simulink model "master_thesis_simulink"  (R2022a)
settings: Solver=VariableStepAuto  StartTime=0.0  StopTime=p_0p.time(end)  FixedStep=0.001  RelTol=1e-3
values from neighbouring files (symbols this model uses):
  markers_forearm = [0.00210510253906 -0.143263397217 -0.00798474121094]    [markers_forearm.mat]
  markers_shoulder = [0.010127746582 -0.151647644043 -0.0119686279297]    [markers_shoulder.mat]
undefined symbols (not defined in the file or in its folder): arm, DiscIntNeverNeededParam, Discrete, ekf, kf, LS, m, markers_hand, n, noise, q0, q0_LS, q0_model, sample_Time, selected, state_observer, Time, tSh_0_0Conf, X, Y, Z
libraries: sm_lib x2029, nesl_utility x1553, robotlib x75, ctrlSharedLib x8
(part 33 of 70)

== system master_thesis_simulink/Ros2Matlab/S1_F1_H2/Subscriber/M3/Pose ==
  Bus : BusSelector  OutputSignals=Pose.Position.X,Pose.Position.Y,Pose.Position.Z
  Mux : Mux  Inputs=3
  Subscribe_pose : robotlib/Subscribe  topicSource=Select from ROS network  topic=/qualisys/Super_marker_3/pose  messageType=geometry_msgs/PoseStamped  SampleTime=sample_Time  legacyBusStruct=off  messageQueueLength=1
  p3_W : Outport
  tag scope: M3_isNew=global
  wires:
  Bus/1 -> Mux/1  "<X>"
  Mux/1 -> p3_W/1
  Subscribe_pose/2 -> Bus/1
  Bus/3 -> Mux/3  "<Z>"
  Bus/2 -> Mux/2  "<Y>"
  Subscribe_pose/1 -> [M3_isNew]

== system master_thesis_simulink/Ros2Matlab/S1_F1_H2/Subscriber/M4/Odom ==
  Bus1 : BusSelector  OutputSignals=Twist.Twist.Linear.X,Twist.Twist.Linear.Y,Twist.Twist.Linear.Z
  Bus2 : BusSelector  OutputSignals=Pose.Covariance
  Bus3 : BusSelector  OutputSignals=Twist.Covariance
  Mux2 : Mux  Inputs=3
  Subscribe_twist : robotlib/Subscribe  topicSource=Select from ROS network  topic=/qualisys/Super_marker_4/odom  messageType=nav_msgs/Odometry  SampleTime=sample_Time  legacyBusStruct=off  messageQueueLength=1
  Terminator3 : Terminator
  v4_W : Outport
  Rp4_W : Outport  Port=2
  Rv4_W : Outport  Port=3
  wires:
  Mux2/1 -> v4_W/1
  Subscribe_twist/1 -> Terminator3/1
  Bus1/2 -> Mux2/2  "<Y>"
  Bus1/1 -> Mux2/1  "<X>"
  Bus1/3 -> Mux2/3  "<Z>"
  Subscribe_twist/2 -> Bus3/1, Bus2/1, Bus1/1
  Bus2/1 -> Rp4_W/1  "<Covariance>"
  Bus3/1 -> Rv4_W/1  "<Covariance>"

== system master_thesis_simulink/Ros2Matlab/S1_F1_H2/Subscriber/M4/Pose ==
  Bus : BusSelector  OutputSignals=Pose.Position.X,Pose.Position.Y,Pose.Position.Z
  Mux : Mux  Inputs=3
  Subscribe_pose : robotlib/Subscribe  topicSource=Select from ROS network  topic=/qualisys/Super_marker_4/pose  messageType=geometry_msgs/PoseStamped  SampleTime=sample_Time  legacyBusStruct=off  messageQueueLength=1
  p4_W : Outport
  tag scope: M4_isNew=global
  wires:
  Bus/2 -> Mux/2  "<Y>"
  Bus/3 -> Mux/3  "<Z>"
  Subscribe_pose/2 -> Bus/1
  Mux/1 -> p4_W/1
  Bus/1 -> Mux/1  "<X>"
  Subscribe_pose/1 -> [M4_isNew]

== system master_thesis_simulink/Ros2Matlab/S1_F1_H2/Subscriber/Shoulder_RF/Pose ==
  Bus Selector : BusSelector  OutputSignals=Pose.Orientation.W
  Bus Selector1 : BusSelector  OutputSignals=Pose.Orientation.X
  Bus Selector2 : BusSelector  OutputSignals=Pose.Orientation.Y
  Bus Selector3 : BusSelector  OutputSignals=Pose.Position.X,Pose.Position.Y,Pose.Position.Z
  Bus Selector4 : BusSelector  OutputSignals=Pose.Orientation.Z
  Mux1 : Mux  Inputs=3
  Mux2 : Mux
  Subscribe_pose : robotlib/Subscribe  topicSource=Select from ROS network  topic=/qualisys/Shoulder_RF/pose  messageType=geometry_msgs/PoseStamped  SampleTime=sample_Time  legacyBusStruct=off  messageQueueLength=1
  quat_Sh2W : Outport
  pSh_W : Outport  Port=2
  tag scope: Sh_isNew=global
  wires:
  Mux2/1 -> quat_Sh2W/1
  Bus Selector4/1 -> Mux2/4  "<Z>"
  Mux1/1 -> pSh_W/1
  Bus Selector3/3 -> Mux1/3  "<Z>"
  Bus Selector3/2 -> Mux1/2  "<Y>"
  Bus Selector3/1 -> Mux1/1  "<X>"
  Bus Selector2/1 -> Mux2/3  "<Y>"
  Bus Selector1/1 -> Mux2/2  "<X>"
  Bus Selector/1 -> Mux2/1  "<W>"
  Subscribe_pose/2 -> Bus Selector/1, Bus Selector1/1, Bus Selector2/1, Bus Selector3/1, Bus Selector4/1
  Subscribe_pose/1 -> [Sh_isNew]

== system master_thesis_simulink/Ros2Matlab/S1_F2_H2/Subscriber/M0/Odom ==
  Bus Selector : BusSelector  OutputSignals=Pose.Covariance
  Bus Selector1 : BusSelector  OutputSignals=Twist.Covariance
  Bus1 : BusSelector  OutputSignals=Twist.Twist.Linear.X,Twist.Twist.Linear.Y,Twist.Twist.Linear.Z
  Mux2 : Mux  Inputs=3
  Subscribe_odom : robotlib/Subscribe  topicSource=Select from ROS network  topic=/qualisys/Super_marker_0/odom  messageType=nav_msgs/Odometry  SampleTime=sample_Time  legacyBusStruct=off  messageQueueLength=1
  Terminator3 : Terminator
  v0_W : Outport
  Rp0_W : Outport  Port=2
  Rv0_W : Outport  Port=3
  wires:
  Bus Selector1/1 -> Rv0_W/1  "<Covariance>"
  Bus Selector/1 -> Rp0_W/1  "<Covariance>"
  Subscribe_odom/2 -> Bus1/1, Bus Selector/1, Bus Selector1/1
  Mux2/1 -> v0_W/1
  Subscribe_odom/1 -> Terminator3/1
  Bus1/2 -> Mux2/2  "<Y>"
  Bus1/1 -> Mux2/1  "<X>"
  Bus1/3 -> Mux2/3  "<Z>"

== system master_thesis_simulink/Ros2Matlab/S1_F2_H2/Subscriber/M0/Pose ==
  Bus Selector : BusSelector  OutputSignals=Pose.Orientation.W
  Bus Selector1 : BusSelector  OutputSignals=Pose.Orientation.X
  Bus Selector2 : BusSelector  OutputSignals=Pose.Orientation.Y
  Bus Selector3 : BusSelector  OutputSignals=Pose.Position.X,Pose.Position.Y,Pose.Position.Z
  Bus Selector4 : BusSelector  OutputSignals=Pose.Orientation.Z
  Mux1 : Mux  Inputs=3
  Mux2 : Mux
  Subscribe_pose : robotlib/Subscribe  topicSource=Select from ROS network  topic=/qualisys/Super_marker_0/pose  messageType=geometry_msgs/PoseStamped  SampleTime=sample_Time  legacyBusStruct=off  messageQueueLength=1
  quat_02W : Outport
  p0_W : Outport  Port=2
  tag scope: M0_isNew=global
  wires:
  Subscribe_pose/1 -> [M0_isNew]
  Subscribe_pose/2 -> Bus Selector4/1, Bus Selector3/1, Bus Selector2/1, Bus Selector1/1, Bus Selector/1
  Bus Selector/1 -> Mux2/1  "<W>"
  Bus Selector1/1 -> Mux2/2  "<X>"
  Bus Selector2/1 -> Mux2/3  "<Y>"
  Bus Selector3/1 -> Mux1/1  "<X>"
  Bus Selector3/2 -> Mux1/2  "<Y>"
  Bus Selector3/3 -> Mux1/3  "<Z>"
  Mux1/1 -> p0_W/1
  Bus Selector4/1 -> Mux2/4  "<Z>"
  Mux2/1 -> quat_02W/1

== system master_thesis_simulink/Ros2Matlab/S1_F2_H2/Subscriber/M1/Odom ==
  Bus1 : BusSelector  OutputSignals=Twist.Twist.Linear.X,Twist.Twist.Linear.Y,Twist.Twist.Linear.Z
  Bus2 : BusSelector  OutputSignals=Pose.Covariance
  Bus3 : BusSelector  OutputSignals=Twist.Covariance
  Mux2 : Mux  Inputs=3
  Subscribe_twist : robotlib/Subscribe  topicSource=Select from ROS network  topic=/qualisys/Super_marker_1/odom  messageType=nav_msgs/Odometry  SampleTime=sample_Time  legacyBusStruct=off  messageQueueLength=1
  Terminator3 : Terminator
  v1_W : Outport
  Rp1_W : Outport  Port=2
  Rv1_W : Outport  Port=3
  wires:
  Bus3/1 -> Rv1_W/1  "<Covariance>"
  Bus2/1 -> Rp1_W/1  "<Covariance>"
  Subscribe_twist/2 -> Bus1/1, Bus2/1, Bus3/1
  Mux2/1 -> v1_W/1
  Subscribe_twist/1 -> Terminator3/1
  Bus1/2 -> Mux2/2  "<Y>"
  Bus1/1 -> Mux2/1  "<X>"
  Bus1/3 -> Mux2/3  "<Z>"

== system master_thesis_simulink/Ros2Matlab/S1_F2_H2/Subscriber/M1/Pose ==
  Bus : BusSelector  OutputSignals=Pose.Position.X,Pose.Position.Y,Pose.Position.Z
  Mux : Mux  Inputs=3
  Subscribe_pose : robotlib/Subscribe  topicSource=Select from ROS network  topic=/qualisys/Super_marker_1/pose  messageType=geometry_msgs/PoseStamped  SampleTime=sample_Time  legacyBusStruct=off  messageQueueLength=1
  p1_W : Outport
  tag scope: M1_isNew=global
  wires:
  Subscribe_pose/1 -> [M1_isNew]
  Bus/2 -> Mux/2  "<Y>"
  Bus/3 -> Mux/3  "<Z>"
  Subscribe_pose/2 -> Bus/1
  Mux/1 -> p1_W/1
  Bus/1 -> Mux/1  "<X>"

== system master_thesis_simulink/Ros2Matlab/S1_F2_H2/Subscriber/M2/Odom ==
  Bus1 : BusSelector  OutputSignals=Twist.Twist.Linear.X,Twist.Twist.Linear.Y,Twist.Twist.Linear.Z
  Bus2 : BusSelector  OutputSignals=Pose.Covariance
  Bus3 : BusSelector  OutputSignals=Twist.Covariance
  Mux2 : Mux  Inputs=3
  Subscribe_twist : robotlib/Subscribe  topicSource=Select from ROS network  topic=/qualisys/Super_marker_2/odom  messageType=nav_msgs/Odometry  SampleTime=sample_Time  legacyBusStruct=off  messageQueueLength=1
  Terminator3 : Terminator
  v2_W : Outport
  Rp2_W : Outport  Port=2
  Rv2_W : Outport  Port=3
  wires:
  Bus3/1 -> Rv2_W/1  "<Covariance>"
  Subscribe_twist/2 -> Bus1/1, Bus2/1, Bus3/1
  Bus2/1 -> Rp2_W/1  "<Covariance>"
  Bus1/3 -> Mux2/3  "<Z>"
  Bus1/1 -> Mux2/1  "<X>"
  Bus1/2 -> Mux2/2  "<Y>"
  Subscribe_twist/1 -> Terminator3/1
  Mux2/1 -> v2_W/1

== system master_thesis_simulink/Ros2Matlab/S1_F2_H2/Subscriber/M2/Pose ==
  Bus : BusSelector  OutputSignals=Pose.Position.X,Pose.Position.Y,Pose.Position.Z
  Mux : Mux  Inputs=3
  Subscribe_pose : robotlib/Subscribe  topicSource=Select from ROS network  topic=/qualisys/Super_marker_2/pose  messageType=geometry_msgs/PoseStamped  SampleTime=sample_Time  legacyBusStruct=off  messageQueueLength=1
  p2_W : Outport
  tag scope: M2_isNew=global
  wires:
  Subscribe_pose/1 -> [M2_isNew]
  Bus/1 -> Mux/1  "<X>"
  Mux/1 -> p2_W/1
  Subscribe_pose/2 -> Bus/1
  Bus/3 -> Mux/3  "<Z>"
  Bus/2 -> Mux/2  "<Y>"

== system master_thesis_simulink/Ros2Matlab/S1_F2_H2/Subscriber/M3/Odom ==
  Bus1 : BusSelector  OutputSignals=Twist.Twist.Linear.X,Twist.Twist.Linear.Y,Twist.Twist.Linear.Z
  Bus2 : BusSelector  OutputSignals=Pose.Covariance
  Bus3 : BusSelector  OutputSignals=Twist.Covariance
  Mux2 : Mux  Inputs=3
  Subscribe_twist : robotlib/Subscribe  topicSource=Select from ROS network  topic=/qualisys/Super_marker_3/odom  messageType=nav_msgs/Odometry  SampleTime=sample_Time  legacyBusStruct=off  messageQueueLength=1
  Terminator3 : Terminator
  v3_W : Outport
  Rp3_W : Outport  Port=2
  Rv3_W : Outport  Port=3
  wires:
  Bus3/1 -> Rv3_W/1  "<Covariance>"
  Subscribe_twist/2 -> Bus1/1, Bus2/1, Bus3/1
  Bus2/1 -> Rp3_W/1  "<Covariance>"
  Mux2/1 -> v3_W/1
  Subscribe_twist/1 -> Terminator3/1
  Bus1/2 -> Mux2/2  "<Y>"
  Bus1/1 -> Mux2/1  "<X>"
  Bus1/3 -> Mux2/3  "<Z>"

== system master_thesis_simulink/Ros2Matlab/S1_F2_H2/Subscriber/M3/Pose ==
  Bus : BusSelector  OutputSignals=Pose.Position.X,Pose.Position.Y,Pose.Position.Z
  Mux : Mux  Inputs=3
  Subscribe_pose : robotlib/Subscribe  topicSource=Select from ROS network  topic=/qualisys/Super_marker_3/pose  messageType=geometry_msgs/PoseStamped  SampleTime=sample_Time  legacyBusStruct=off  messageQueueLength=1
  p3_W : Outport
  tag scope: M3_isNew=global
  wires:
  Subscribe_pose/1 -> [M3_isNew]
  Bus/2 -> Mux/2  "<Y>"
  Bus/3 -> Mux/3  "<Z>"
  Subscribe_pose/2 -> Bus/1
  Mux/1 -> p3_W/1
  Bus/1 -> Mux/1  "<X>"

== system master_thesis_simulink/Ros2Matlab/S1_F2_H2/Subscriber/M4/Odom ==
  Bus1 : BusSelector  OutputSignals=Twist.Twist.Linear.X,Twist.Twist.Linear.Y,Twist.Twist.Linear.Z
  Bus2 : BusSelector  OutputSignals=Pose.Covariance
  Bus3 : BusSelector  OutputSignals=Twist.Covariance
  Mux2 : Mux  Inputs=3
  Subscribe_twist : robotlib/Subscribe  topicSource=Select from ROS network  topic=/qualisys/Super_marker_4/odom  messageType=nav_msgs/Odometry  SampleTime=sample_Time  legacyBusStruct=off  messageQueueLength=1
  Terminator3 : Terminator
  v4_W : Outport
  Rp4_W : Outport  Port=2
  Rv4_W : Outport  Port=3
  wires:
  Bus3/1 -> Rv4_W/1  "<Covariance>"
  Bus2/1 -> Rp4_W/1  "<Covariance>"
  Subscribe_twist/2 -> Bus1/1, Bus2/1, Bus3/1
  Bus1/3 -> Mux2/3  "<Z>"
  Bus1/1 -> Mux2/1  "<X>"
  Bus1/2 -> Mux2/2  "<Y>"
  Subscribe_twist/1 -> Terminator3/1
  Mux2/1 -> v4_W/1

== system master_thesis_simulink/Ros2Matlab/S1_F2_H2/Subscriber/M4/Pose ==
  Bus : BusSelector  OutputSignals=Pose.Position.X,Pose.Position.Y,Pose.Position.Z
  Mux : Mux  Inputs=3
  Subscribe_pose : robotlib/Subscribe  topicSource=Select from ROS network  topic=/qualisys/Super_marker_4/pose  messageType=geometry_msgs/PoseStamped  SampleTime=sample_Time  legacyBusStruct=off  messageQueueLength=1
  p4_W : Outport
  tag scope: M4_isNew=global
  wires:
  Subscribe_pose/1 -> [M4_isNew]
  Bus/1 -> Mux/1  "<X>"
  Mux/1 -> p4_W/1
  Subscribe_pose/2 -> Bus/1
  Bus/3 -> Mux/3  "<Z>"
  Bus/2 -> Mux/2  "<Y>"

== system master_thesis_simulink/Ros2Matlab/S1_F2_H2/Subscriber/M5/Odom ==
  Bus1 : BusSelector  OutputSignals=Twist.Twist.Linear.X,Twist.Twist.Linear.Y,Twist.Twist.Linear.Z
  Bus2 : BusSelector  OutputSignals=Pose.Covariance
  Bus3 : BusSelector  OutputSignals=Twist.Covariance
  Mux2 : Mux  Inputs=3
  Subscribe_twist : robotlib/Subscribe  topicSource=Select from ROS network  topic=/qualisys/Super_marker_5/odom  messageType=nav_msgs/Odometry  SampleTime=sample_Time  legacyBusStruct=off  messageQueueLength=1
  Terminator3 : Terminator
  v2_W : Outport
  Rp2_W : Outport  Port=2
  Rv2_W : Outport  Port=3
  wires:
  Mux2/1 -> v2_W/1
  Subscribe_twist/1 -> Terminator3/1
  Bus1/2 -> Mux2/2  "<Y>"
  Bus1/1 -> Mux2/1  "<X>"
  Bus1/3 -> Mux2/3  "<Z>"
  Bus2/1 -> Rp2_W/1  "<Covariance>"
  Subscribe_twist/2 -> Bus3/1, Bus2/1, Bus1/1
  Bus3/1 -> Rv2_W/1  "<Covariance>"

== system master_thesis_simulink/Ros2Matlab/S1_F2_H2/Subscriber/M5/Pose ==
  Bus : BusSelector  OutputSignals=Pose.Position.X,Pose.Position.Y,Pose.Position.Z
  Mux : Mux  Inputs=3
  Subscribe_pose : robotlib/Subscribe  topicSource=Select from ROS network  topic=/qualisys/Super_marker_5/pose  messageType=geometry_msgs/PoseStamped  SampleTime=sample_Time  legacyBusStruct=off  messageQueueLength=1
  p5_W : Outport
  tag scope: M5_isNew=global
  wires:
  Bus/2 -> Mux/2  "<Y>"
  Bus/3 -> Mux/3  "<Z>"
  Subscribe_pose/2 -> Bus/1
  Mux/1 -> p5_W/1
  Bus/1 -> Mux/1  "<X>"
  Subscribe_pose/1 -> [M5_isNew]

== system master_thesis_simulink/Ros2Matlab/S1_F2_H2/Subscriber/Shoulder_RF/Pose ==
  Bus Selector : BusSelector  OutputSignals=Pose.Orientation.W
  Bus Selector1 : BusSelector  OutputSignals=Pose.Orientation.X
  Bus Selector2 : BusSelector  OutputSignals=Pose.Orientation.Y
  Bus Selector3 : BusSelector  OutputSignals=Pose.Position.X,Pose.Position.Y,Pose.Position.Z
  Bus Selector4 : BusSelector  OutputSignals=Pose.Orientation.Z
  Mux1 : Mux  Inputs=3
  Mux2 : Mux
  Subscribe_pose : robotlib/Subscribe  topicSource=Select from ROS network  topic=/qualisys/Shoulder_RF/pose  messageType=geometry_msgs/PoseStamped  SampleTime=sample_Time  legacyBusStruct=off  messageQueueLength=1
  quat_Sh2W : Outport
  pSh_W : Outport  Port=2
  tag scope: Sh_isNew=global
  wires:
  Subscribe_pose/1 -> [Sh_isNew]
  Subscribe_pose/2 -> Bus Selector4/1, Bus Selector3/1, Bus Selector2/1, Bus Selector1/1, Bus Selector/1
  Bus Selector/1 -> Mux2/1  "<W>"
  Bus Selector1/1 -> Mux2/2  "<X>"
  Bus Selector2/1 -> Mux2/3  "<Y>"
  Bus Selector3/1 -> Mux1/1  "<X>"
  Bus Selector3/2 -> Mux1/2  "<Y>"
  Bus Selector3/3 -> Mux1/3  "<Z>"
  Mux1/1 -> pSh_W/1
  Bus Selector4/1 -> Mux2/4  "<Z>"
  Mux2/1 -> quat_Sh2W/1

== system master_thesis_simulink/Ros2Matlab/S2_F0_H2/Subscriber/M0/Odom ==
  Bus Selector : BusSelector  OutputSignals=Pose.Covariance
  Bus Selector1 : BusSelector  OutputSignals=Twist.Covariance
  Bus1 : BusSelector  OutputSignals=Twist.Twist.Linear.X,Twist.Twist.Linear.Y,Twist.Twist.Linear.Z
  Mux2 : Mux  Inputs=3
  Subscribe_odom : robotlib/Subscribe  topicSource=Select from ROS network  topic=/qualisys/Super_marker_0/odom  messageType=nav_msgs/Odometry  SampleTime=sample_Time  legacyBusStruct=off  messageQueueLength=1
  Terminator3 : Terminator
  v0_W : Outport
  Rp0_W : Outport  Port=2
  Rv0_W : Outport  Port=3
  wires:
  Bus1/3 -> Mux2/3  "<Z>"
  Bus1/1 -> Mux2/1  "<X>"
  Bus1/2 -> Mux2/2  "<Y>"
  Subscribe_odom/1 -> Terminator3/1
  Mux2/1 -> v0_W/1
  Subscribe_odom/2 -> Bus Selector1/1, Bus Selector/1, Bus1/1
  Bus Selector/1 -> Rp0_W/1  "<Covariance>"
  Bus Selector1/1 -> Rv0_W/1  "<Covariance>"

== system master_thesis_simulink/Ros2Matlab/S2_F0_H2/Subscriber/M0/Pose ==
  Bus Selector : BusSelector  OutputSignals=Pose.Orientation.W
  Bus Selector1 : BusSelector  OutputSignals=Pose.Orientation.X
  Bus Selector2 : BusSelector  OutputSignals=Pose.Orientation.Y
  Bus Selector3 : BusSelector  OutputSignals=Pose.Position.X,Pose.Position.Y,Pose.Position.Z
  Bus Selector4 : BusSelector  OutputSignals=Pose.Orientation.Z
  Mux1 : Mux  Inputs=3
  Mux2 : Mux
  Subscribe_pose : robotlib/Subscribe  topicSource=Select from ROS network  topic=/qualisys/Super_marker_0/pose  messageType=geometry_msgs/PoseStamped  SampleTime=sample_Time  legacyBusStruct=off  messageQueueLength=1
  quat_02W : Outport
  p0_W : Outport  Port=2
  tag scope: M0_isNew=global
  wires:
  Mux2/1 -> quat_02W/1
  Bus Selector4/1 -> Mux2/4  "<Z>"
  Mux1/1 -> p0_W/1
  Bus Selector3/3 -> Mux1/3  "<Z>"
  Bus Selector3/2 -> Mux1/2  "<Y>"
  Bus Selector3/1 -> Mux1/1  "<X>"
  Bus Selector2/1 -> Mux2/3  "<Y>"
  Bus Selector1/1 -> Mux2/2  "<X>"
  Bus Selector/1 -> Mux2/1  "<W>"
  Subscribe_pose/2 -> Bus Selector/1, Bus Selector1/1, Bus Selector2/1, Bus Selector3/1, Bus Selector4/1
  Subscribe_pose/1 -> [M0_isNew]

== system master_thesis_simulink/Ros2Matlab/S2_F0_H2/Subscriber/M1/Odom ==
  Bus1 : BusSelector  OutputSignals=Twist.Twist.Linear.X,Twist.Twist.Linear.Y,Twist.Twist.Linear.Z
  Bus2 : BusSelector  OutputSignals=Pose.Covariance
  Bus3 : BusSelector  OutputSignals=Twist.Covariance
  Mux2 : Mux  Inputs=3
  Subscribe_twist : robotlib/Subscribe  topicSource=Select from ROS network  topic=/qualisys/Super_marker_1/odom  messageType=nav_msgs/Odometry  SampleTime=sample_Time  legacyBusStruct=off  messageQueueLength=1
  Terminator3 : Terminator
  v1_W : Outport
  Rp1_W : Outport  Port=2
  Rv1_W : Outport  Port=3
  wires:
  Bus1/3 -> Mux2/3  "<Z>"
  Bus1/1 -> Mux2/1  "<X>"
  Bus1/2 -> Mux2/2  "<Y>"
  Subscribe_twist/1 -> Terminator3/1
  Mux2/1 -> v1_W/1
  Subscribe_twist/2 -> Bus3/1, Bus2/1, Bus1/1
  Bus2/1 -> Rp1_W/1  "<Covariance>"
  Bus3/1 -> Rv1_W/1  "<Covariance>"

== system master_thesis_simulink/Ros2Matlab/S2_F0_H2/Subscriber/M1/Pose ==
  Bus : BusSelector  OutputSignals=Pose.Position.X,Pose.Position.Y,Pose.Position.Z
  Mux : Mux  Inputs=3
  Subscribe_pose : robotlib/Subscribe  topicSource=Select from ROS network  topic=/qualisys/Super_marker_1/pose  messageType=geometry_msgs/PoseStamped  SampleTime=sample_Time  legacyBusStruct=off  messageQueueLength=1
  p1_W : Outport
  tag scope: M1_isNew=global
  wires:
  Bus/1 -> Mux/1  "<X>"
  Mux/1 -> p1_W/1
  Subscribe_pose/2 -> Bus/1
  Bus/3 -> Mux/3  "<Z>"
  Bus/2 -> Mux/2  "<Y>"
  Subscribe_pose/1 -> [M1_isNew]

== system master_thesis_simulink/Ros2Matlab/S2_F0_H2/Subscriber/M2/Odom ==
  Bus1 : BusSelector  OutputSignals=Twist.Twist.Linear.X,Twist.Twist.Linear.Y,Twist.Twist.Linear.Z
  Bus2 : BusSelector  OutputSignals=Pose.Covariance
  Bus3 : BusSelector  OutputSignals=Twist.Covariance
  Mux2 : Mux  Inputs=3
  Subscribe_twist : robotlib/Subscribe  topicSource=Select from ROS network  topic=/qualisys/Super_marker_2/odom  messageType=nav_msgs/Odometry  SampleTime=sample_Time  legacyBusStruct=off  messageQueueLength=1
  Terminator3 : Terminator
  v2_W : Outport
  Rp2_W : Outport  Port=2
  Rv2_W : Outport  Port=3
  wires:
  Mux2/1 -> v2_W/1
  Subscribe_twist/1 -> Terminator3/1
  Bus1/2 -> Mux2/2  "<Y>"
  Bus1/1 -> Mux2/1  "<X>"
  Bus1/3 -> Mux2/3  "<Z>"
  Bus2/1 -> Rp2_W/1  "<Covariance>"
  Subscribe_twist/2 -> Bus3/1, Bus2/1, Bus1/1
  Bus3/1 -> Rv2_W/1  "<Covariance>"

== system master_thesis_simulink/Ros2Matlab/S2_F0_H2/Subscriber/M2/Pose ==
  Bus : BusSelector  OutputSignals=Pose.Position.X,Pose.Position.Y,Pose.Position.Z
  Mux : Mux  Inputs=3
  Subscribe_pose : robotlib/Subscribe  topicSource=Select from ROS network  topic=/qualisys/Super_marker_2/pose  messageType=geometry_msgs/PoseStamped  SampleTime=sample_Time  legacyBusStruct=off  messageQueueLength=1
  p2_W : Outport
  tag scope: M2_isNew=global
  wires:
  Bus/2 -> Mux/2  "<Y>"
  Bus/3 -> Mux/3  "<Z>"
  Subscribe_pose/2 -> Bus/1
  Mux/1 -> p2_W/1
  Bus/1 -> Mux/1  "<X>"
  Subscribe_pose/1 -> [M2_isNew]

== system master_thesis_simulink/Ros2Matlab/S2_F0_H2/Subscriber/M3/Odom ==
  Bus1 : BusSelector  OutputSignals=Twist.Twist.Linear.X,Twist.Twist.Linear.Y,Twist.Twist.Linear.Z
  Bus2 : BusSelector  OutputSignals=Pose.Covariance
  Bus3 : BusSelector  OutputSignals=Twist.Covariance
  Mux2 : Mux  Inputs=3
  Subscribe_twist : robotlib/Subscribe  topicSource=Select from ROS network  topic=/qualisys/Super_marker_3/odom  messageType=nav_msgs/Odometry  SampleTime=sample_Time  legacyBusStruct=off  messageQueueLength=1
  Terminator3 : Terminator
  v3_W : Outport
  Rp3_W : Outport  Port=2
  Rv3_W : Outport  Port=3
  wires:
  Bus1/3 -> Mux2/3  "<Z>"
  Bus1/1 -> Mux2/1  "<X>"
  Bus1/2 -> Mux2/2  "<Y>"
  Subscribe_twist/1 -> Terminator3/1
  Mux2/1 -> v3_W/1
  Bus2/1 -> Rp3_W/1  "<Covariance>"
  Subscribe_twist/2 -> Bus3/1, Bus2/1, Bus1/1
  Bus3/1 -> Rv3_W/1  "<Covariance>"

== system master_thesis_simulink/Ros2Matlab/S2_F0_H2/Subscriber/M3/Pose ==
  Bus : BusSelector  OutputSignals=Pose.Position.X,Pose.Position.Y,Pose.Position.Z
  Mux : Mux  Inputs=3
  Subscribe_pose : robotlib/Subscribe  topicSource=Select from ROS network  topic=/qualisys/Super_marker_3/pose  messageType=geometry_msgs/PoseStamped  SampleTime=sample_Time  legacyBusStruct=off  messageQueueLength=1
  p3_W : Outport
  tag scope: M3_isNew=global
  wires:
  Bus/1 -> Mux/1  "<X>"
  Mux/1 -> p3_W/1
  Subscribe_pose/2 -> Bus/1
  Bus/3 -> Mux/3  "<Z>"
  Bus/2 -> Mux/2  "<Y>"
  Subscribe_pose/1 -> [M3_isNew]

== system master_thesis_simulink/Ros2Matlab/S2_F0_H2/Subscriber/M4/Odom ==
  Bus1 : BusSelector  OutputSignals=Twist.Twist.Linear.X,Twist.Twist.Linear.Y,Twist.Twist.Linear.Z
  Bus2 : BusSelector  OutputSignals=Pose.Covariance
  Bus3 : BusSelector  OutputSignals=Twist.Covariance
  Mux2 : Mux  Inputs=3
  Subscribe_twist : robotlib/Subscribe  topicSource=Select from ROS network  topic=/qualisys/Super_marker_4/odom  messageType=nav_msgs/Odometry  SampleTime=sample_Time  legacyBusStruct=off  messageQueueLength=1
  Terminator3 : Terminator
  v4_W : Outport
  Rp4_W : Outport  Port=2
  Rv4_W : Outport  Port=3
  wires:
  Mux2/1 -> v4_W/1
  Subscribe_twist/1 -> Terminator3/1
  Bus1/2 -> Mux2/2  "<Y>"
  Bus1/1 -> Mux2/1  "<X>"
  Bus1/3 -> Mux2/3  "<Z>"
  Subscribe_twist/2 -> Bus3/1, Bus2/1, Bus1/1
  Bus2/1 -> Rp4_W/1  "<Covariance>"
  Bus3/1 -> Rv4_W/1  "<Covariance>"

== system master_thesis_simulink/Ros2Matlab/S2_F0_H2/Subscriber/M4/Pose ==
  Bus : BusSelector  OutputSignals=Pose.Position.X,Pose.Position.Y,Pose.Position.Z
  Mux : Mux  Inputs=3
  Subscribe_pose : robotlib/Subscribe  topicSource=Select from ROS network  topic=/qualisys/Super_marker_4/pose  messageType=geometry_msgs/PoseStamped  SampleTime=sample_Time  legacyBusStruct=off  messageQueueLength=1
  p4_W : Outport
  tag scope: M4_isNew=global
  wires:
  Bus/2 -> Mux/2  "<Y>"
  Bus/3 -> Mux/3  "<Z>"
  Subscribe_pose/2 -> Bus/1
  Mux/1 -> p4_W/1
  Bus/1 -> Mux/1  "<X>"
  Subscribe_pose/1 -> [M4_isNew]

== system master_thesis_simulink/Ros2Matlab/S2_F0_H2/Subscriber/Shoulder_RF/Pose ==
  Bus Selector : BusSelector  OutputSignals=Pose.Orientation.W
  Bus Selector1 : BusSelector  OutputSignals=Pose.Orientation.X
  Bus Selector2 : BusSelector  OutputSignals=Pose.Orientation.Y
  Bus Selector3 : BusSelector  OutputSignals=Pose.Position.X,Pose.Position.Y,Pose.Position.Z
  Bus Selector4 : BusSelector  OutputSignals=Pose.Orientation.Z
  Mux1 : Mux  Inputs=3
  Mux2 : Mux
  Subscribe_pose : robotlib/Subscribe  topicSource=Select from ROS network  topic=/qualisys/Shoulder_RF/pose  messageType=geometry_msgs/PoseStamped  SampleTime=sample_Time  legacyBusStruct=off  messageQueueLength=1
  quat_Sh2W : Outport
  pSh_W : Outport  Port=2
  tag scope: Sh_isNew=global
  wires:
  Mux2/1 -> quat_Sh2W/1
  Bus Selector4/1 -> Mux2/4  "<Z>"
  Mux1/1 -> pSh_W/1
  Bus Selector3/3 -> Mux1/3  "<Z>"
  Bus Selector3/2 -> Mux1/2  "<Y>"
  Bus Selector3/1 -> Mux1/1  "<X>"
  Bus Selector2/1 -> Mux2/3  "<Y>"
  Bus Selector1/1 -> Mux2/2  "<X>"
  Bus Selector/1 -> Mux2/1  "<W>"
  Subscribe_pose/2 -> Bus Selector/1, Bus Selector1/1, Bus Selector2/1, Bus Selector3/1, Bus Selector4/1
  Subscribe_pose/1 -> [Sh_isNew]

== system master_thesis_simulink/System/Human arm/RightHand/Markers/M1 ==
  Marker 1 : sm_lib/Body Elements/Spherical Solid  GraphicAmbientColor=[0.15 0.15 0.15 1.0]  BasedOnType=Density  CenterOfMass=[0 0 0]  CenterOfMassUnits=m  GraphicDiffuseColor=[1.0 0.2 0.2]  Density=1000  DensityUnits=kg/m^3  DoExposeReferenceFrame=on  GraphicEmissiveColor=[0.0 0.0 0.0 1.0]  ExportEntireGeometry=off  SerializedExposedGeometries=<ExposedGeometries/>  SerializedFrames=<Frames/>  MarkerShape=Sphere  MarkerSize=10  GraphicType=FromGeometry  InertiaType=CalculateFromGeometry  Mass=1  MassUnits=kg  MomentsOfInertia=[1 1 1]  MomentsOfInertiaUnits=kg*m^2  GraphicOpacity=1.0  ProductsOfInertia=[0 0 0]  ProductsOfInertiaUnits=kg*m^2  GraphicShininess=75  GraphicSpecularColor=[0.5 0.5 0.5 1.0]  SphereRadius=arm.markers.radius  SphereRadiusUnits=m  GraphicVisPropType=SimpleVisualProperties
  Mux11 : Mux  Inputs=3
  Mux3 : Mux  Inputs=3
  PS-Simulink Converter{9..11,34..36} (6 alike) : nesl_utility/PS-Simulink Converter  PhysicalDomain=network_engine_domain  SubClassName=ps_output  LeftPortType=input  RightPortType=output  PseudoPeriodic=off  Frequencies=[]  VectorFormat=inherit  Unit=inherit  AffineConversion=off
      settings: SourceProductBaseCode=SS,PW,VE
  Transform Sensor3 : sm_lib/Frames and Transforms/Transform Sensor  MeasurementFrame=World  SenseAngle=off  SenseAxis=off  SenseAngle1=off  SenseAngle2=off  SenseAngle3=off  SenseQ=off  SenseR=off  SenseOmegaX=off  SenseOmegaY=off  SenseOmegaZ=off  SenseOmega1=off  SenseOmega2=off  SenseOmega3=off  SenseQDot=off  SenseRDot=off  SenseAlphaX=off  SenseAlphaY=off  SenseAlphaZ=off  SenseAlpha1=off  SenseAlpha2=off  SenseAlpha3=off  SenseQDDot=off  SenseRDDot=off  SenseX=on  SenseY=on  SenseZ=on  SenseRad=off  SenseAzim=off  SenseDist=off  SenseInc=off  SenseXDot=on  SenseYDot=on  SenseZDot=on  SenseRadDot=off  SenseAzimDot=off  SenseDistDot=off  SenseIncDot=off  SenseXDDot=off  SenseYDDot=off  SenseZDDot=off  SenseRadDDot=off  SenseAzimDDot=off  SenseDistDDot=off  SenseIncDDot=off
  translation_R2Base : sm_lib/Frames and Transforms/Rigid Transform  TranslationMethod=Cartesian  TranslationStandardOffset=0  TranslationLengthUnit=m  TranslationStandardAxis=+Z  TranslationCartesianOffset=[0 arm.hand.dimensions(2)/2 0]  TranslationROffset=0  TranslationROffsetUnits=m  TranslationZOffset=0  TranslationZOffsetUnits=m  TranslationThetaOffset=0  TranslationThetaOffsetUnits=deg  RotationMethod=None  RotationAngleUnits=rad  RotationStandardAxis=+Z  RotationAngle=pi/2  RotationArbitraryAxis=[1 0 0]  FollAlignAxisA=+X  BaseAlignAxisA=+Y  FollAlignAxisB=+Y  BaseAlignAxisB=+Z  RotationSequenceAxes=BaseAxes  RotationSequence=XYZ  RotationSequenceAngles=[pi/2, 0, 0]  RotationSequenceAnglesUnits=rad  RotationMatrix=[1 0 0; 0 1 0; 0 0 1]
  translation_x : sm_lib/Frames and Transforms/Rigid Transform  TranslationMethod=Cartesian  TranslationStandardOffset=0  TranslationLengthUnit=m  TranslationStandardAxis=+Z  TranslationCartesianOffset=[markers_hand(1,1) 0 0]  TranslationROffset=0  TranslationROffsetUnits=m  TranslationZOffset=0  TranslationZOffsetUnits=m  TranslationThetaOffset=0  TranslationThetaOffsetUnits=deg  RotationMethod=None  RotationAngleUnits=rad  RotationStandardAxis=+Z  RotationAngle=pi/2  RotationArbitraryAxis=[1 0 0]  FollAlignAxisA=+X  BaseAlignAxisA=+Y  FollAlignAxisB=+Y  BaseAlignAxisB=+Z  RotationSequenceAxes=BaseAxes  RotationSequence=XYZ  RotationSequenceAngles=[pi/2, 0, 0]  RotationSequenceAnglesUnits=rad  RotationMatrix=[1 0 0; 0 1 0; 0 0 1]
  translation_y : sm_lib/Frames and Transforms/Rigid Transform  TranslationMethod=Cartesian  TranslationStandardOffset=0  TranslationLengthUnit=m  TranslationStandardAxis=+Z  TranslationCartesianOffset=[0 markers_hand(2,1) 0]  TranslationROffset=0  TranslationROffsetUnits=m  TranslationZOffset=0  TranslationZOffsetUnits=m  TranslationThetaOffset=0  TranslationThetaOffsetUnits=deg  RotationMethod=None  RotationAngleUnits=rad  RotationStandardAxis=+Z  RotationAngle=pi/2  RotationArbitraryAxis=[1 0 0]  FollAlignAxisA=+X  BaseAlignAxisA=+Y  FollAlignAxisB=+Y  BaseAlignAxisB=+Z  RotationSequenceAxes=BaseAxes  RotationSequence=XYZ  RotationSequenceAngles=[pi/2, 0, 0]  RotationSequenceAnglesUnits=rad  RotationMatrix=[1 0 0; 0 1 0; 0 0 1]
  translation_z : sm_lib/Frames and Transforms/Rigid Transform  TranslationMethod=Cartesian  TranslationStandardOffset=0  TranslationLengthUnit=m  TranslationStandardAxis=+Z  TranslationCartesianOffset=[0 0 markers_hand(3,1)]  TranslationROffset=0  TranslationROffsetUnits=m  TranslationZOffset=0  TranslationZOffsetUnits=m  TranslationThetaOffset=0  TranslationThetaOffsetUnits=deg  RotationMethod=None  RotationAngleUnits=rad  RotationStandardAxis=+Z  RotationAngle=pi/2  RotationArbitraryAxis=[1 0 0]  FollAlignAxisA=+X  BaseAlignAxisA=+Y  FollAlignAxisB=+Y  BaseAlignAxisB=+Z  RotationSequenceAxes=BaseAxes  RotationSequence=XYZ  RotationSequenceAngles=[pi/2, 0, 0]  RotationSequenceAnglesUnits=rad  RotationMatrix=[1 0 0; 0 1 0; 0 0 1]
  W : PMIOPort  Side=Left
  R : PMIOPort  Port=2  Side=Left
  p_1 : Outport
  pdot_1 : Outport  Port=2
  wires:
  PS-Simulink Converter36/1 -> Mux3/3  "M1_posz"
  PS-Simulink Converter34/1 -> Mux3/1  "M1_posx"
  PS-Simulink Converter11/1 -> Mux11/3  "M1_velz"
  Mux3/1 -> p_1/1
  PS-Simulink Converter10/1 -> Mux11/2  "M1_vely"
  PS-Simulink Converter35/1 -> Mux3/2  "M1_posy"
  PS-Simulink Converter9/1 -> Mux11/1  "M1_velx"
  Mux11/1 -> pdot_1/1
  connections:
  translation_z/RConn1 -- Transform Sensor3/RConn1 -- Marker 1/RConn1
  translation_R2Base/RConn1 -- translation_x/LConn1
  translation_R2Base/LConn1 -- R/RConn1
  translation_y/LConn1 -- translation_x/RConn1
  Transform Sensor3/RConn4 -- PS-Simulink Converter36/LConn1
  PS-Simulink Converter35/LConn1 -- Transform Sensor3/RConn3
  W/RConn1 -- Transform Sensor3/LConn1
  translation_z/LConn1 -- translation_y/RConn1
  PS-Simulink Converter10/LConn1 -- Transform Sensor3/RConn6
  PS-Simulink Converter11/LConn1 -- Transform Sensor3/RConn7
  PS-Simulink Converter34/LConn1 -- Transform Sensor3/RConn2
  PS-Simulink Converter9/LConn1 -- Transform Sensor3/RConn5

== system master_thesis_simulink/System/Human arm/RightHand/Markers/M2 ==
  Marker 1 : sm_lib/Body Elements/Spherical Solid  GraphicAmbientColor=[0.15 0.15 0.15 1.0]  BasedOnType=Density  CenterOfMass=[0 0 0]  CenterOfMassUnits=m  GraphicDiffuseColor=[1.0 0.2 0.2]  Density=1000  DensityUnits=kg/m^3  DoExposeReferenceFrame=on  GraphicEmissiveColor=[0.0 0.0 0.0 1.0]  ExportEntireGeometry=off  SerializedExposedGeometries=<ExposedGeometries/>  SerializedFrames=<Frames/>  MarkerShape=Sphere  MarkerSize=10  GraphicType=FromGeometry  InertiaType=CalculateFromGeometry  Mass=1  MassUnits=kg  MomentsOfInertia=[1 1 1]  MomentsOfInertiaUnits=kg*m^2  GraphicOpacity=1.0  ProductsOfInertia=[0 0 0]  ProductsOfInertiaUnits=kg*m^2  GraphicShininess=75  GraphicSpecularColor=[0.5 0.5 0.5 1.0]  SphereRadius=arm.markers.radius  SphereRadiusUnits=m  GraphicVisPropType=SimpleVisualProperties
  Mux11 : Mux  Inputs=3
  Mux3 : Mux  Inputs=3
  PS-Simulink Converter{9..11,34..36} (6 alike) : nesl_utility/PS-Simulink Converter  PhysicalDomain=network_engine_domain  SubClassName=ps_output  LeftPortType=input  RightPortType=output  PseudoPeriodic=off  Frequencies=[]  VectorFormat=inherit  Unit=inherit  AffineConversion=off
      settings: SourceProductBaseCode=SS,PW,VE
  Transform Sensor3 : sm_lib/Frames and Transforms/Transform Sensor  MeasurementFrame=World  SenseAngle=off  SenseAxis=off  SenseAngle1=off  SenseAngle2=off  SenseAngle3=off  SenseQ=off  SenseR=off  SenseOmegaX=off  SenseOmegaY=off  SenseOmegaZ=off  SenseOmega1=off  SenseOmega2=off  SenseOmega3=off  SenseQDot=off  SenseRDot=off  SenseAlphaX=off  SenseAlphaY=off  SenseAlphaZ=off  SenseAlpha1=off  SenseAlpha2=off  SenseAlpha3=off  SenseQDDot=off  SenseRDDot=off  SenseX=on  SenseY=on  SenseZ=on  SenseRad=off  SenseAzim=off  SenseDist=off  SenseInc=off  SenseXDot=on  SenseYDot=on  SenseZDot=on  SenseRadDot=off  SenseAzimDot=off  SenseDistDot=off  SenseIncDot=off  SenseXDDot=off  SenseYDDot=off  SenseZDDot=off  SenseRadDDot=off  SenseAzimDDot=off  SenseDistDDot=off  SenseIncDDot=off
  translation_R2Base : sm_lib/Frames and Transforms/Rigid Transform  TranslationMethod=Cartesian  TranslationStandardOffset=0  TranslationLengthUnit=m  TranslationStandardAxis=+Z  TranslationCartesianOffset=[0 arm.hand.dimensions(2)/2 0]  TranslationROffset=0  TranslationROffsetUnits=m  TranslationZOffset=0  TranslationZOffsetUnits=m  TranslationThetaOffset=0  TranslationThetaOffsetUnits=deg  RotationMethod=None  RotationAngleUnits=rad  RotationStandardAxis=+Z  RotationAngle=pi/2  RotationArbitraryAxis=[1 0 0]  FollAlignAxisA=+X  BaseAlignAxisA=+Y  FollAlignAxisB=+Y  BaseAlignAxisB=+Z  RotationSequenceAxes=BaseAxes  RotationSequence=XYZ  RotationSequenceAngles=[pi/2, 0, 0]  RotationSequenceAnglesUnits=rad  RotationMatrix=[1 0 0; 0 1 0; 0 0 1]
  translation_x : sm_lib/Frames and Transforms/Rigid Transform  TranslationMethod=Cartesian  TranslationStandardOffset=0  TranslationLengthUnit=m  TranslationStandardAxis=+Z  TranslationCartesianOffset=[markers_hand(1,2) 0 0]  TranslationROffset=0  TranslationROffsetUnits=m  TranslationZOffset=0  TranslationZOffsetUnits=m  TranslationThetaOffset=0  TranslationThetaOffsetUnits=deg  RotationMethod=None  RotationAngleUnits=rad  RotationStandardAxis=+Z  RotationAngle=pi/2  RotationArbitraryAxis=[1 0 0]  FollAlignAxisA=+X  BaseAlignAxisA=+Y  FollAlignAxisB=+Y  BaseAlignAxisB=+Z  RotationSequenceAxes=BaseAxes  RotationSequence=XYZ  RotationSequenceAngles=[pi/2, 0, 0]  RotationSequenceAnglesUnits=rad  RotationMatrix=[1 0 0; 0 1 0; 0 0 1]
  translation_y : sm_lib/Frames and Transforms/Rigid Transform  TranslationMethod=Cartesian  TranslationStandardOffset=0  TranslationLengthUnit=m  TranslationStandardAxis=+Z  TranslationCartesianOffset=[0 markers_hand(2,2) 0]  TranslationROffset=0  TranslationROffsetUnits=m  TranslationZOffset=0  TranslationZOffsetUnits=m  TranslationThetaOffset=0  TranslationThetaOffsetUnits=deg  RotationMethod=None  RotationAngleUnits=rad  RotationStandardAxis=+Z  RotationAngle=pi/2  RotationArbitraryAxis=[1 0 0]  FollAlignAxisA=+X  BaseAlignAxisA=+Y  FollAlignAxisB=+Y  BaseAlignAxisB=+Z  RotationSequenceAxes=BaseAxes  RotationSequence=XYZ  RotationSequenceAngles=[pi/2, 0, 0]  RotationSequenceAnglesUnits=rad  RotationMatrix=[1 0 0; 0 1 0; 0 0 1]
  translation_z : sm_lib/Frames and Transforms/Rigid Transform  TranslationMethod=Cartesian  TranslationStandardOffset=0  TranslationLengthUnit=m  TranslationStandardAxis=+Z  TranslationCartesianOffset=[0 0 markers_hand(3,2)]  TranslationROffset=0  TranslationROffsetUnits=m  TranslationZOffset=0  TranslationZOffsetUnits=m  TranslationThetaOffset=0  TranslationThetaOffsetUnits=deg  RotationMethod=None  RotationAngleUnits=rad  RotationStandardAxis=+Z  RotationAngle=pi/2  RotationArbitraryAxis=[1 0 0]  FollAlignAxisA=+X  BaseAlignAxisA=+Y  FollAlignAxisB=+Y  BaseAlignAxisB=+Z  RotationSequenceAxes=BaseAxes  RotationSequence=XYZ  RotationSequenceAngles=[pi/2, 0, 0]  RotationSequenceAnglesUnits=rad  RotationMatrix=[1 0 0; 0 1 0; 0 0 1]
  W : PMIOPort  Side=Left
  R : PMIOPort  Port=2  Side=Left
  p_1 : Outport
  pdot_1 : Outport  Port=2
  wires:
  Mux11/1 -> pdot_1/1
  PS-Simulink Converter9/1 -> Mux11/1  "M1_velx"
  PS-Simulink Converter35/1 -> Mux3/2  "M1_posy"
  PS-Simulink Converter10/1 -> Mux11/2  "M1_vely"
  Mux3/1 -> p_1/1
  PS-Simulink Converter11/1 -> Mux11/3  "M1_velz"
  PS-Simulink Converter34/1 -> Mux3/1  "M1_posx"
  PS-Simulink Converter36/1 -> Mux3/3  "M1_posz"
  connections:
  PS-Simulink Converter9/LConn1 -- Transform Sensor3/RConn5
  PS-Simulink Converter34/LConn1 -- Transform Sensor3/RConn2
  PS-Simulink Converter11/LConn1 -- Transform Sensor3/RConn7
  PS-Simulink Converter10/LConn1 -- Transform Sensor3/RConn6
  translation_z/LConn1 -- translation_y/RConn1
  W/RConn1 -- Transform Sensor3/LConn1
  PS-Simulink Converter35/LConn1 -- Transform Sensor3/RConn3
  Transform Sensor3/RConn4 -- PS-Simulink Converter36/LConn1
  translation_y/LConn1 -- translation_x/RConn1
  translation_R2Base/LConn1 -- R/RConn1
  translation_R2Base/RConn1 -- translation_x/LConn1
  Marker 1/RConn1 -- Transform Sensor3/RConn1 -- translation_z/RConn1

== system master_thesis_simulink/System/Human arm/RightShoulder/Markers/M1 ==
  Marker 1 : sm_lib/Body Elements/Spherical Solid  GraphicAmbientColor=[0.15 0.15 0.15 1.0]  BasedOnType=Density  CenterOfMass=[0 0 0]  CenterOfMassUnits=m  GraphicDiffuseColor=[1.0 0.2 0.2]  Density=1000  DensityUnits=kg/m^3  DoExposeReferenceFrame=on  GraphicEmissiveColor=[0.0 0.0 0.0 1.0]  ExportEntireGeometry=off  SerializedExposedGeometries=<ExposedGeometries/>  SerializedFrames=<Frames/>  MarkerShape=Sphere  MarkerSize=10  GraphicType=FromGeometry  InertiaType=CalculateFromGeometry  Mass=1  MassUnits=kg  MomentsOfInertia=[1 1 1]  MomentsOfInertiaUnits=kg*m^2  GraphicOpacity=1.0  ProductsOfInertia=[0 0 0]  ProductsOfInertiaUnits=kg*m^2  GraphicShininess=75  GraphicSpecularColor=[0.5 0.5 0.5 1.0]  SphereRadius=arm.markers.radius  SphereRadiusUnits=m  GraphicVisPropType=SimpleVisualProperties
  Mux11 : Mux  Inputs=3
  Mux3 : Mux  Inputs=3
  PS-Simulink Converter{9..11,34..36} (6 alike) : nesl_utility/PS-Simulink Converter  PhysicalDomain=network_engine_domain  SubClassName=ps_output  LeftPortType=input  RightPortType=output  PseudoPeriodic=off  Frequencies=[]  VectorFormat=inherit  Unit=inherit  AffineConversion=off
      settings: SourceProductBaseCode=SS,PW,VE
  Transform Sensor3 : sm_lib/Frames and Transforms/Transform Sensor  MeasurementFrame=World  SenseAngle=off  SenseAxis=off  SenseAngle1=off  SenseAngle2=off  SenseAngle3=off  SenseQ=off  SenseR=off  SenseOmegaX=off  SenseOmegaY=off  SenseOmegaZ=off  SenseOmega1=off  SenseOmega2=off  SenseOmega3=off  SenseQDot=off  SenseRDot=off  SenseAlphaX=off  SenseAlphaY=off  SenseAlphaZ=off  SenseAlpha1=off  SenseAlpha2=off  SenseAlpha3=off  SenseQDDot=off  SenseRDDot=off  SenseX=on  SenseY=on  SenseZ=on  SenseRad=off  SenseAzim=off  SenseDist=off  SenseInc=off  SenseXDot=on  SenseYDot=on  SenseZDot=on  SenseRadDot=off  SenseAzimDot=off  SenseDistDot=off  SenseIncDot=off  SenseXDDot=off  SenseYDDot=off  SenseZDDot=off  SenseRadDDot=off  SenseAzimDDot=off  SenseDistDDot=off  SenseIncDDot=off
  translation_R2Base : sm_lib/Frames and Transforms/Rigid Transform  TranslationMethod=Cartesian  TranslationStandardOffset=0  TranslationLengthUnit=m  TranslationStandardAxis=+Z  TranslationCartesianOffset=[0 arm.shoulder.length/2 0]  TranslationROffset=0  TranslationROffsetUnits=m  TranslationZOffset=0  TranslationZOffsetUnits=m  TranslationThetaOffset=0  TranslationThetaOffsetUnits=deg  RotationMethod=None  RotationAngleUnits=rad  RotationStandardAxis=+Z  RotationAngle=pi/2  RotationArbitraryAxis=[1 0 0]  FollAlignAxisA=+X  BaseAlignAxisA=+Y  FollAlignAxisB=+Y  BaseAlignAxisB=+Z  RotationSequenceAxes=BaseAxes  RotationSequence=XYZ  RotationSequenceAngles=[pi/2, 0, 0]  RotationSequenceAnglesUnits=rad  RotationMatrix=[1 0 0; 0 1 0; 0 0 1]
  translation_x : sm_lib/Frames and Transforms/Rigid Transform  TranslationMethod=Cartesian  TranslationStandardOffset=0  TranslationLengthUnit=m  TranslationStandardAxis=+Z  TranslationCartesianOffset=[markers_shoulder(1,1) 0 0]  TranslationROffset=0  TranslationROffsetUnits=m  TranslationZOffset=0  TranslationZOffsetUnits=m  TranslationThetaOffset=0  TranslationThetaOffsetUnits=deg  RotationMethod=None  RotationAngleUnits=rad  RotationStandardAxis=+Z  RotationAngle=pi/2  RotationArbitraryAxis=[1 0 0]  FollAlignAxisA=+X  BaseAlignAxisA=+Y  FollAlignAxisB=+Y  BaseAlignAxisB=+Z  RotationSequenceAxes=BaseAxes  RotationSequence=XYZ  RotationSequenceAngles=[pi/2, 0, 0]  RotationSequenceAnglesUnits=rad  RotationMatrix=[1 0 0; 0 1 0; 0 0 1]
  translation_y : sm_lib/Frames and Transforms/Rigid Transform  TranslationMethod=Cartesian  TranslationStandardOffset=0  TranslationLengthUnit=m  TranslationStandardAxis=+Z  TranslationCartesianOffset=[0 markers_shoulder(2,1) 0]  TranslationROffset=0  TranslationROffsetUnits=m  TranslationZOffset=0  TranslationZOffsetUnits=m  TranslationThetaOffset=0  TranslationThetaOffsetUnits=deg  RotationMethod=None  RotationAngleUnits=rad  RotationStandardAxis=+Z  RotationAngle=pi/2  RotationArbitraryAxis=[1 0 0]  FollAlignAxisA=+X  BaseAlignAxisA=+Y  FollAlignAxisB=+Y  BaseAlignAxisB=+Z  RotationSequenceAxes=BaseAxes  RotationSequence=XYZ  RotationSequenceAngles=[pi/2, 0, 0]  RotationSequenceAnglesUnits=rad  RotationMatrix=[1 0 0; 0 1 0; 0 0 1]
  translation_z : sm_lib/Frames and Transforms/Rigid Transform  TranslationMethod=Cartesian  TranslationStandardOffset=0  TranslationLengthUnit=m  TranslationStandardAxis=+Z  TranslationCartesianOffset=[0 0 markers_shoulder(3,1)]  TranslationROffset=0  TranslationROffsetUnits=m  TranslationZOffset=0  TranslationZOffsetUnits=m  TranslationThetaOffset=0  TranslationThetaOffsetUnits=deg  RotationMethod=None  RotationAngleUnits=rad  RotationStandardAxis=+Z  RotationAngle=pi/2  RotationArbitraryAxis=[1 0 0]  FollAlignAxisA=+X  BaseAlignAxisA=+Y  FollAlignAxisB=+Y  BaseAlignAxisB=+Z  RotationSequenceAxes=BaseAxes  RotationSequence=XYZ  RotationSequenceAngles=[pi/2, 0, 0]  RotationSequenceAnglesUnits=rad  RotationMatrix=[1 0 0; 0 1 0; 0 0 1]
  W : PMIOPort  Side=Left
  R : PMIOPort  Port=2  Side=Left
  p_1 : Outport
  pdot_1 : Outport  Port=2
  wires:
  PS-Simulink Converter36/1 -> Mux3/3  "M1_posz"
  PS-Simulink Converter34/1 -> Mux3/1  "M1_posx"
  PS-Simulink Converter11/1 -> Mux11/3  "M1_velz"
  Mux3/1 -> p_1/1
  PS-Simulink Converter10/1 -> Mux11/2  "M1_vely"
  PS-Simulink Converter35/1 -> Mux3/2  "M1_posy"
  PS-Simulink Converter9/1 -> Mux11/1  "M1_velx"
  Mux11/1 -> pdot_1/1
  connections:
  translation_z/RConn1 -- Transform Sensor3/RConn1 -- Marker 1/RConn1
  translation_R2Base/RConn1 -- translation_x/LConn1
  translation_R2Base/LConn1 -- R/RConn1
  translation_y/LConn1 -- translation_x/RConn1
  Transform Sensor3/RConn4 -- PS-Simulink Converter36/LConn1
  PS-Simulink Converter35/LConn1 -- Transform Sensor3/RConn3
  W/RConn1 -- Transform Sensor3/LConn1
  translation_z/LConn1 -- translation_y/RConn1
  PS-Simulink Converter10/LConn1 -- Transform Sensor3/RConn6
  PS-Simulink Converter11/LConn1 -- Transform Sensor3/RConn7
  PS-Simulink Converter34/LConn1 -- Transform Sensor3/RConn2
  PS-Simulink Converter9/LConn1 -- Transform Sensor3/RConn5

== system master_thesis_simulink/System/Show Results/EKF/Human arm/Elbow_joint ==
  Input : Inport
  Constant : Constant  Value=pi/6
  Signal Generator1 : SignalGenerator  Amplitude=pi/7  Frequency=1.2*pi  Units=rad/sec
  Signal Generator3 : SignalGenerator  Amplitude=pi/9  Frequency=pi  Units=rad/sec
  Sum : Sum  Inputs=|++-
  c1 : nesl_utility/Simulink-PS Converter  PhysicalDomain=network_engine_domain  SubClassName=ps_input  LeftPortType=input  RightPortType=output  PseudoPeriodic=off  Frequencies=[]  NoiseDistribution=none  NoiseParameters=[]  Unit=1  AffineConversion=off  FilteringAndDerivatives=filter  SimscapeFilterOrder=2  InputFilterTimeConstant=0.001  UdotUserProvided=0
      settings: SourceProductBaseCode=SS,PW,VE
  jRightElbow_rotx : sm_lib/Joints/Revolute Joint  JointMode=Normal  SenseConstraintForce=off  SenseConstraintForceX=off  SenseConstraintForceY=off  SenseConstraintForceZ=off  SenseConstraintTorque=off  SenseConstraintTorqueX=off  SenseConstraintTorqueY=off  SenseConstraintTorqueZ=off  SenseTotalForce=off  SenseTotalForceX=off  SenseTotalForceY=off  SenseTotalForceZ=off  SenseTotalTorque=off  SenseTotalTorqueX=off  SenseTotalTorqueY=off  SenseTotalTorqueZ=off  CompositeWrenchDir=FollowerOnBase  CompositeWrenchFrame=BaseFrame  EquilibriumPosition=0  EquilibriumPositionUnits=deg  SpringStiffness=0  SpringStiffnessUnits=N*m/deg  DampingCoefficient=0.1  DampingCoefficientUnits=kg*m^2/(rad*s)  TorqueActuationMode=ComputedTorque  MotionActuationMode=InputMotion  SensePosition=on  SenseVelocity=on  SenseAcceleration=off  SenseTorqueForce=off  SenseLowerLimitTorqueForce=off  SenseUpperLimitTorqueForce=off  LowerLimitSpecify=on  LowerLimitBound=-3/4*pi  LowerLimitBoundUnits=rad  LowerLimitStiffness=1e4  LowerLimitStiffnessUnits=N*m/deg  LowerLimitDamping=10  LowerLimitDampingUnits=N*m/(deg/s)  LowerLimitTransitionRegionWidth=0.1  LowerLimitTransitionRegionWidthUnits=deg  UpperLimitSpecify=on  UpperLimitBound=0  UpperLimitBoundUnits=rad  UpperLimitStiffness=1e4  UpperLimitStiffnessUnits=N*m/deg  UpperLimitDamping=10  UpperLimitDampingUnits=N*m/(deg/s)  UpperLimitTransitionRegionWidth=0.1  UpperLimitTransitionRegionWidthUnits=deg  PositionTargetSpecify=off  PositionTargetPriority=Low  PositionTargetValue=0  PositionTargetValueUnits=rad  VelocityTargetSpecify=off  VelocityTargetPriority=High  VelocityTargetValue=0  VelocityTargetValueUnits=deg/s
  B_elbow : PMIOPort  Side=Right
  F_shoulder : PMIOPort  Port=2  Side=Left
  wires:
  Constant/1 -> Sum/1
  Signal Generator3/1 -> Sum/2
  Signal Generator1/1 -> Sum/3
  Input/1 -> c1/1
  connections:
  ?
  ?
  ?
  F_shoulder/RConn1 -- jRightElbow_rotx/LConn1
  jRightElbow_rotx/RConn1 -- B_elbow/RConn1
  c1/RConn1 -- jRightElbow_rotx/LConn2

== system master_thesis_simulink/System/Show Results/EKF/Human arm/Markers ==
  M1 : Subsystem
  W : PMIOPort  Side=Left
  R : PMIOPort  Port=2  Side=Left
  tag scope: p=global, pdot=global
  wires:
  M1/1(p_1) -> [p]
  M1/2(pdot_1) -> [pdot]
  connections:
  R/RConn1 -- M1/LConn2
  W/RConn1 -- M1/LConn1
